simulink model "pendulum"  (R2018a)
settings: Solver=VariableStepAuto  StartTime=0.0  StopTime=ttotal  RelTol=1e-8
values from neighbouring files (symbols this model uses):
  g = 9.8    [e_32.m]    (also in e_34.m; e_34b.m; lab1.m; matlab.mat)
  l = 0.5    [e_32.m]    (also in e_34.m; e_34b.m; lab1.m; matlab.mat)
  m = 30    [e_15.m]    (also in e_32.m = 1; e_34.m = 1; e_34b.m = 1; lab1.m = 1)
  p10 = 0    [e_32.m]    (also in e_34.m = p0_calc(1); e_34b.m = p0_calc(1); lab1.m = p0_calc(1); matlab.mat = -0.0654498469498)
  p20 = 0    [e_32.m]    (also in e_34.m = p0_calc(2); e_34b.m = p0_calc(2); lab1.m = p0_calc(2); matlab.mat = -0.0436332312999)
  t10 = t10_sim(n)    [e_32.m]    (also in e_34.m = t0_calc(1); e_34b.m = t0_calc(1); lab1.m = t0_calc(1); matlab.mat = nan)
  t20 = t20_sim(n)    [e_32.m]    (also in e_34.m = t0_calc(2); e_34b.m = t0_calc(2); lab1.m = t0_calc(2); matlab.mat = nan)
settings Model: Creator=root  LastModifiedBy=root

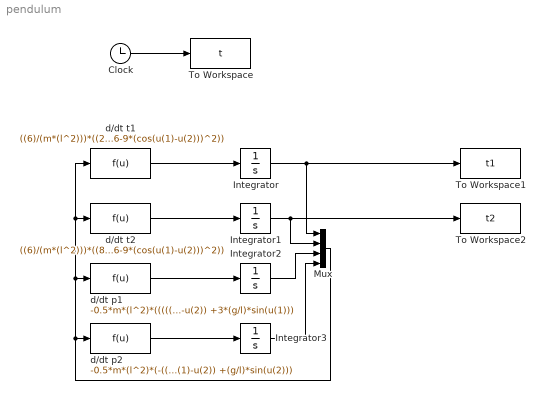
== system pendulum ==
  Clock : Clock
  Integrator : Integrator  InitialCondition=t10
  Integrator1 : Integrator  InitialCondition=t20
  Integrator2 : Integrator  InitialCondition=p10
  Integrator3 : Integrator  InitialCondition=p20
  Mux : Mux
  To Workspace : ToWorkspace  VariableName=t  SampleTime=-1
  To Workspace1 : ToWorkspace  VariableName=t1  SampleTime=-1
  To Workspace2 : ToWorkspace  VariableName=t2  SampleTime=-1
  d/dt p1 : Fcn  Expr=-0.5*m*(l^2)*(((((6)/(m*(l^2)))*((2*u(3)-3*cos(u(1)-u(2))*u(4))/(16-9*(cos(u(1)-u(2)))^2)))*(((6)/(m*(l^2)))*((8*u(4)-3*cos(u(1)-u(2))*u(3))/(16-9*(cos(u(1)-u(2)))^2))))*sin(u(1)-u(2)) +3*(g/l)*sin(u(1)))
  d/dt p2 : Fcn  Expr=-0.5*m*(l^2)*(-((((6)/(m*(l^2)))*((2*u(3)-3*cos(u(1)-u(2))*u(4))/(16-9*(cos(u(1)-u(2)))^2)))*(((6)/(m*(l^2)))*((8*u(4)-3*cos(u(1)-u(2))*u(3))/(16-9*(cos(u(1)-u(2)))^2))))*sin(u(1)-u(2)) +(g/l)*sin(u(2)))
  d/dt t1 : Fcn  Expr=((6)/(m*(l^2)))*((2*u(3)-3*cos(u(1)-u(2))*u(4))/(16-9*(cos(u(1)-u(2)))^2))
  d/dt t2 : Fcn  Expr=((6)/(m*(l^2)))*((8*u(4)-3*cos(u(1)-u(2))*u(3))/(16-9*(cos(u(1)-u(2)))^2))
  wires:
  d/dt t1/1 -> Integrator/1
  d/dt t2/1 -> Integrator1/1
  d/dt p1/1 -> Integrator2/1
  d/dt p2/1 -> Integrator3/1
  Integrator/1 -> To Workspace1/1, Mux/1
  Integrator1/1 -> To Workspace2/1, Mux/2
  Integrator2/1 -> Mux/3
  Integrator3/1 -> Mux/4
  Mux/1 -> d/dt p2/1, d/dt t1/1, d/dt t2/1, d/dt p1/1
  Clock/1 -> To Workspace/1
